simulink model "generic_nlp_ocp_solver_simulink_block"  (R2024b)
settings: Solver=FixedStepDiscrete  StartTime=0.0  StopTime=inf  FixedStep=0.002  RelTol=1e-3  EnableMultiTasking=on
undefined symbols (not defined in the file or in its folder): HIL
libraries: quarc_library x3
settings Model: ExtModeTrigDuration=10000  Creator=dinhck  LastModifiedBy=dinhck
settings SolverCC: AlgebraicLoopSolver=TrustRegion  PositivePriorityOrder=on  AutoInsertRateTranBlk=on
settings DataIOCC: ReturnWorkspaceOutputs=off
settings DebuggingCC: UnconnectedInputMsg=warning  UnconnectedOutputMsg=warning  UnconnectedLineMsg=warning  ArithmeticOperatorsInVariantConditions=warning
settings ModelReferenceCC: EnableRefExpFcnMdlSchedulingChecks=on
settings SFSimCC: SimUseLocalCustomCode=off  CustomCodeUndefinedFunction=UseInterfaceOnly
settings RTWCC: Description=QUARC Win64 Target Using Toolchain  SystemTargetFile=quarc_win64.tlc  TemplateMakefile=quarc_default_tmf  RTWUseLocalCustomCode=off  Toolchain=QUARC win64 | nmake (64-bit Windows)  BuildConfiguration=Faster Runs  GPUComputeCapability=3.5
settings RTWCC: CustomInclude=|
  | "C:\Users\dinhck\deps\acados\include"
  | "C:\Users\dinhck\deps\acados\include\acados_c"
  | "C:\Users\dinhck\deps\acados\include\blasfeo\include"
  | "C:\Users\dinhck\deps\acados\include\hpipm\include"
settings RTWCC: CustomSource=|
  | "C:\Users\dinhck\dev\project\quanser_dc_motor\acados_dc_motor\c_generated_code\acados_solver_generic_nlp.c"
  | "C:\Users\dinhck\dev\project\quanser_dc_motor\acados_dc_motor\c_generated_code\generic_nlp_constraints\generic_nlp_constr_h_e_fun.c"
  | "C:\Users\dinhck\dev\project\quanser_dc_motor\acados_dc_motor\c_generated_code\generic_nlp_constraints\generic_nlp_constr_h_e_fun_jac_uxt_zt.c"
  | "C:\Users\dinhck\dev\project\quanser_dc_motor\acados_dc_motor\c_generated_code\generic_nlp_cost\generic_nlp_cost_ext_cost_e_fun.c"
  | "C:\Users\dinhck\dev\project\quanser_dc_motor\acados_dc_motor\c_generated_code\generic_nlp_cost\generic_nlp_cost_ext_cost_e_fun_jac.c"
  | "C:\Users\dinhck\dev\project\quanser_dc_motor\acados_dc_motor\c_generated_code\generic_nlp_cost\generic_nlp_cost_ext_cost_e_fun_jac_hess.c"
settings RTWCC: CustomLibrary=|
  | "C:\Users\dinhck\deps\acados\lib\acados.lib"
  | "C:\Users\dinhck\deps\acados\lib\blasfeo.lib"
  | "C:\Users\dinhck\deps\acados\lib\hpipm.lib"
  | "C:\Users\dinhck\deps\acados\lib\osqp.lib"
  | "C:\Users\dinhck\deps\acados\lib\qpOASES_e.lib"
settings CodeAppCC: StateflowObjectComments=on
settings STFCustomTargetCC: TargetLangStandard=C99 (ISO)  ConcurrentExecutionCompliant=on  GRTInterface=on  UseToolchainInfoCompliant=on  SystemTargetFile=quarc_win64.tlc
settings GRTTargetCC: ParMdlRefBuildCompliant=off  CompOptLevelCompliant=off  CombineOutputUpdateFcns=off  MatFileLogging=off  CPPClassGenCompliant=off  GRTInterface=on  ExtMode=on  ExtModeMexFile=quarc_comm
settings ConfigComp: CovMetricSettings=dswe

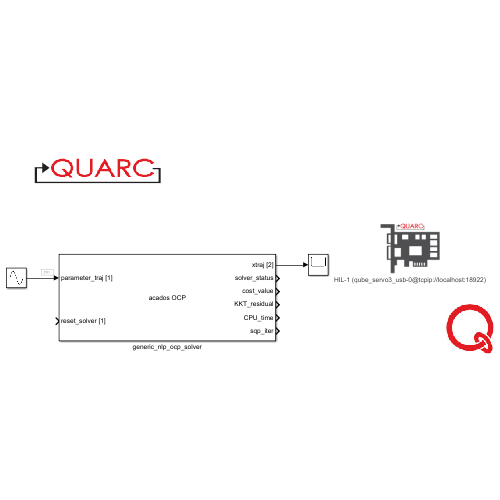
[thumbnail: Simulink's stored preview of the top-level diagram]
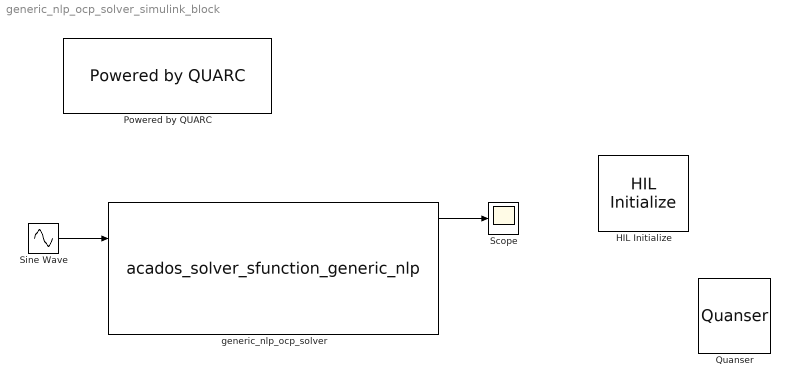
== system generic_nlp_ocp_solver_simulink_block ==
  HIL Initialize : quarc_library/Data Acquisition/Generic/Configuration/HIL Initialize  object_name=HIL-1  board_type=qube_servo3_usb  board_number=0@tcpip://localhost:18922  board_options=deadband_compensation=0.3;pwm_en=0;enc0_velocity=3.0;enc1_velocity=3.0;min_diode_compensation=0.3;max_diode_compensation=1.5  exclusive=off  active=on  hardware_clocks=[0]  clock_modes=[]  initial_clock_frequencies=[]  set_clock_params_at_start=off  set_clock_params_at_switch_in=off  set_clock_frequencies_at_start=off  set_clock_frequencies_at_switch_in=off  analog_input_channels=[0]  analog_input_configurations=[]  analog_input_maximums=3  analog_input_minimums=-3  set_analog_input_params_at_start=off  set_analog_input_params_at_switch_in=off  analog_output_channels=[0]  analog_output_maximums=15  analog_output_minimums=-15  initial_analog_outputs=[0]  final_analog_outputs=[0]  watchdog_analog_outputs=0  set_analog_output_params_at_start=off  set_analog_output_params_at_switch_in=off  set_analog_outputs_at_start=on  set_analog_outputs_at_switch_in=off  set_analog_outputs_at_terminate=on  set_analog_outputs_at_switch_out=off  set_analog_outputs_on_watchdog=on  digital_input_channels=[]  digital_output_channels=[0]  digital_output_configuration=[]  initial_digital_outputs=[1]  final_digital_outputs=[0]  watchdog_digital_outputs=[0]  set_digital_output_params_at_start=off  set_digital_output_params_at_switch_in=off  set_digital_outputs_at_start=on  set_digital_outputs_at_switch_in=off  set_digital_outputs_at_terminate=on  set_digital_outputs_at_switch_out=off  set_digital_outputs_on_watchdog=on  encoder_channels=[0:1]  quadrature=[4]  encoder_filter_frequency=[]  initial_encoder_counts=[0]  set_encoder_params_at_start=off  set_encoder_params_at_switch_in=off  set_encoder_counts_at_start=on  set_encoder_counts_at_switch_in=off  pwm_channels=[]  pwm_modes=[0]  pwm_frequency=23195  pwm_configuration=[1]  pwm_alignment=[0]  pwm_polarity=[1]  pwm_leading_deadband=[0]  pwm_trailing_deadband=[0]  initial_pwm_outputs=[0]  final_pwm_outputs=[0]  watchdog_pwm_outputs=[]  set_pwm_params_at_start=off  set_pwm_params_at_switch_in=off  set_pwm_outputs_at_start=off  set_pwm_outputs_at_switch_in=off  set_pwm_outputs_at_terminate=off  set_pwm_outputs_at_switch_out=off  set_pwm_outputs_on_watchdog=off  other_output_channels=[11000:11002]  initial_other_outputs=[0 1 0]  final_other_outputs=[1 0 0]  watchdog_other_outputs=[0 0 1]  set_other_outputs_at_start=on  set_other_outputs_at_switch_in=off  set_other_outputs_at_terminate=on  set_other_outputs_at_switch_out=off  set_other_outputs_on_watchdog=on
  Powered by QUARC : quarc_library/Logos/Powered by QUARC
  Quanser : quarc_library/Logos/Quanser
  Scope : Scope
  Sine Wave : Sin  Amplitude=1.5  Bias=1.5  SampleTime=0
  generic_nlp_ocp_solver : S-Function  FunctionName=acados_solver_sfunction_generic_nlp  SFunctionDeploymentMode=off  EnableBusSupport=off
      mask Display:
      | global sfun_input_names sfun_output_names
      | for i = 1:length(sfun_input_names)
      |     port_label('input', i, sfun_input_names{i})
      | end
      | for i = 1:length(sfun_output_names)
      |     port_label('output', i, sfun_output_names{i})
      | end
      | disp("acados OCP")
  wires:
  Sine Wave/1 -> generic_nlp_ocp_solver/1
  generic_nlp_ocp_solver/1 -> Scope/1
